simulink model "autosar_swc_throttle_sensor"  (R2021a)
settings: Solver=FixedStepDiscrete  StartTime=0.0  StopTime=10.0  FixedStep=0.005  RelTol=1e-3
model workspace (MATLAB code in the model file):
  | TPSPercent_LkupTbl = Simulink.LookupTable;
  | TPSPercent_LkupTbl.Table.DataType = 'single';
  | TPSPercent_LkupTbl.Table.Min = [];
  | TPSPercent_LkupTbl.Table.Max = [];
  | TPSPercent_LkupTbl.Table.Unit = '';
  | TPSPercent_LkupTbl.Table.FieldName = 'Table';
  | TPSPercent_LkupTbl.Table.Description = '';
  | TPSPercent_LkupTbl.Table.Value = ...
  |   [0 10 20 30 40 50 60 70 80 90 100];
  | TPSPercent_LkupTbl.BreakpointsSpecification = 'Explicit values';
  | TPSPercent_LkupTbl.SupportTunableSize = false;
  | TPSPercent_LkupTbl.Breakpoints.DataType = 'single';
  | TPSPercent_LkupTbl.Breakpoints.Min = [];
  | TPSPercent_LkupTbl.Breakpoints.Max = [];
  | TPSPercent_LkupTbl.Breakpoints.Unit = '';
  | TPSPercent_LkupTbl.Breakpoints.FieldName = 'BP1';
  | TPSPercent_LkupTbl.Breakpoints.Description = '';
  | TPSPercent_LkupTbl.Breakpoints.Value = single(linspace(170, 966, 11));
  | TPSPercent_LkupTbl.Breakpoints.TunableSizeName = 'N1';
  | TPSPercent_LkupTbl.CoderInfo.StorageClass = 'Auto';
  | TPSPercent_LkupTbl.StructTypeInfo.Name = 'MyStruct';
  | TPSPercent_LkupTbl.StructTypeInfo.DataScope = 'Auto';
  | TPSPercent_LkupTbl.StructTypeInfo.HeaderFileName = 'Rte_Type.h';
undefined symbols (not defined in the file): TPSPercentBkpt, TPSPercentTbl
settings Model: ParameterArgumentNames=TPSPercent_LkupTbl1  OrderedModelArguments=off  Creator=The MathWorks, Inc.  LastModifiedBy=ASUS
settings SolverCC: AlgebraicLoopSolver=TrustRegion
settings DataIOCC: SaveFormat=StructureWithTime  ReturnWorkspaceOutputs=off
settings OptimizationCC: DefaultParameterBehavior=Inlined  PassReuseOutputArgsAs=Individual arguments  ZeroExternalMemoryAtStartup=off  ZeroInternalMemoryAtStartup=off  EfficientTunableParamExpr=on
settings DebuggingCC: ParameterTunabilityLossMsg=error  SFMachineParentedDataDiag=warning  ArithmeticOperatorsInVariantConditions=warning
settings SFSimCC: SimUseLocalCustomCode=off  MATLABDynamicMemAlloc=off  CustomCodeUndefinedFunction=UseInterfaceOnly
settings RTWCC: Description=AUTOSAR  SystemTargetFile=autosar.tlc  GenCodeOnly=on  TemplateMakefile=ert_default_tmf  GenerateReport=on  RTWUseLocalCustomCode=off  IncludeHyperlinkInReport=on  LaunchReport=on  GenerateTraceInfo=on  GenerateTraceReport=on  GenerateTraceReportSl=on  GenerateTraceReportSf=on  GenerateTraceReportEml=on
settings CodeAppCC: ForceParamTrailComments=on  IgnoreCustomStorageClasses=off  OperatorAnnotations=on  SimulinkDataObjDesc=on  SFDataObjDesc=on  InsertBlockDesc=on
settings STFCustomTargetCC: TargetLangStandard=C99 (ISO)  MultiwordLength=256  ParMdlRefBuildCompliant=on  CompOptLevelCompliant=on  IncludeMdlTerminateFcn=off  CombineOutputUpdateFcns=on  SuppressErrorStatus=on  ERTCustomFileBanners=on  CodeInterfacePackaging=Reusable function  SupportNonFinite=off  SupportComplex=off  SupportContinuousTime=off  SupportNonInlinedSFcns=off  RemoveResetFunc=on  MATLABClassNameForMDSCustomization=Simulink.SoftwareTarget.ERTCustomization  CPPClassGenCompliant=on  AutosarCompliant=on  GRTInterface=off  LookupTableObjectStructAxisOrder=2,1,3,4,...  LUTObjectStructOrderEvenSpacing=Size,Table,Breakpoints  SystemTargetFile=autosar.tlc
settings ERTTargetCC: TargetLangStandard=C99 (ISO)  ConcurrentExecutionCompliant=off  IncludeMdlTerminateFcn=off  SuppressErrorStatus=on  CodeInterfacePackaging=Reusable function  SupportNonFinite=off  SupportComplex=off  ModelStepFunctionPrototypeControlCompliant=off  AutosarCompliant=on  LookupTableObjectStructAxisOrder=2,1,3,4,...  LUTObjectStructOrderEvenSpacing=Size,Table,Breakpoints  InlinedParameterPlacement=NonHierarchical  ERTCustomFileTemplate=example_file_process.tlc

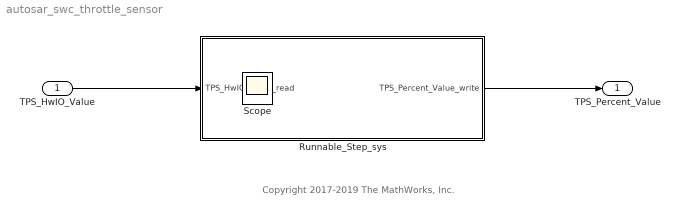
== system autosar_swc_throttle_sensor ==
  note: Copyright 2017-2019 The MathWorks, Inc.
  TPS_HwIO_Value : Inport  OutDataTypeStr=uint16  PortDimensions=1
  Runnable_Step_sys : Subsystem  TreatAsAtomicUnit=on  SystemSampleTime=0.005
  TPS_Percent_Value : Outport  OutDataTypeStr=single  PortDimensions=1  VectorParamsAs1DForOutWhenUnconnected=off
  Scope : Scope
  wires:
  TPS_HwIO_Value/1 -> Runnable_Step_sys/1(TPS_HwIO_Value_read)
  Runnable_Step_sys/1(TPS_Percent_Value_write) -> TPS_Percent_Value/1

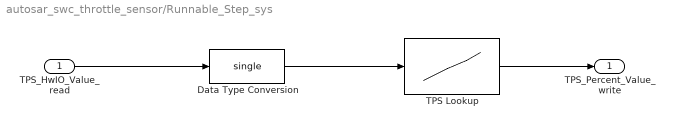
== system autosar_swc_throttle_sensor/Runnable_Step_sys ==
  TPS_HwIO_Value_read : Inport
  Data Type Conversion : DataTypeConversion  OutDataTypeStr=single
  TPS Lookup : Lookup_n-D  NumberOfTableDimensions=1  DataSpecification=Lookup table object  LookupTableObject=TPSPercent_LkupTbl  BreakpointsForDimension1=TPSPercentBkpt  BreakpointsForDimension1DataTypeStr=single  IndexSearchMethod=Linear search  Table=TPSPercentTbl  TableDataTypeStr=single  ExtrapMethod=Clip  InternalRulePriority=Speed  OutDataTypeStr=single  RndMeth=Simplest  InputSameDT=on
  TPS_Percent_Value_write : Outport  VectorParamsAs1DForOutWhenUnconnected=off
  wires:
  TPS_HwIO_Value_read/1 -> Data Type Conversion/1
  TPS Lookup/1 -> TPS_Percent_Value_write/1
  Data Type Conversion/1 -> TPS Lookup/1
